simulink model "Glide_slope_model"  (R2020a)
settings: Solver=VariableStepAuto  StartTime=0.0  StopTime=130  RelTol=1e-3
undefined symbols (not defined in the file): med_AA, med_BB, med_CC, med_DD, trim_control_lo
settings Model: Creator=mathi  LastModifiedBy=mathi

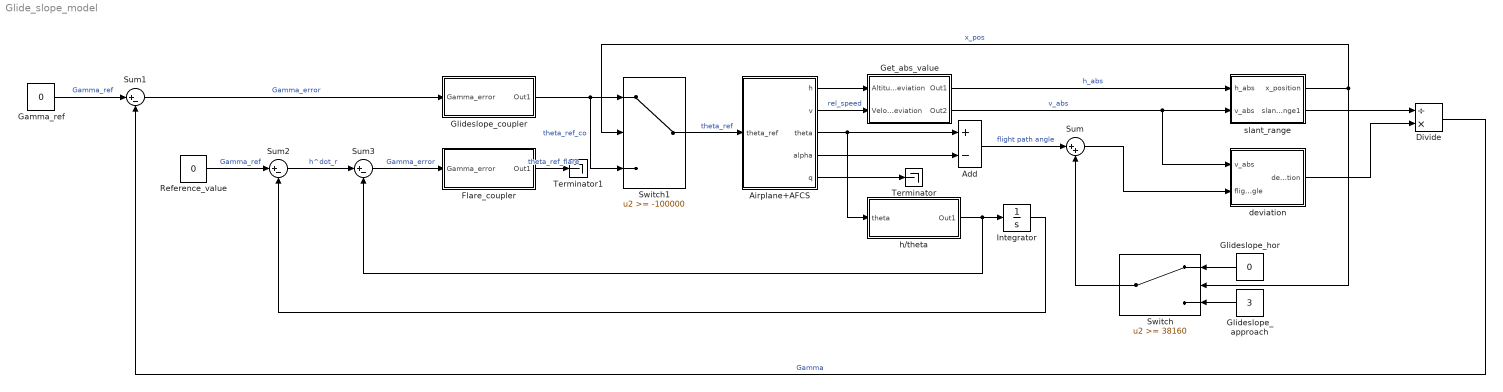
== system Glide_slope_model ==
  Add : Sum  Inputs=+-
  Airplane+AFCS : Subsystem
  Divide : Product  Inputs=/*
  Flare_coupler : Subsystem
  Gamma_ref : Constant  Value=0
  Get_abs_value : Subsystem
  Glideslope_approach : Constant  Value=3
  Glideslope_coupler : Subsystem
  Glideslope_hor : Constant  Value=0
  Integrator : Integrator
  Reference_value : Constant  Value=0
  Sum : Sum  Inputs=|++
  Sum1 : Sum  Inputs=|+-
  Sum2 : Sum  Inputs=|+-
  Sum3 : Sum  Inputs=|+-
  Switch : Switch  Threshold=38160
  Switch1 : Switch  Threshold=-100000
  Terminator : Terminator
  Terminator1 : Terminator
  deviation : Subsystem
  h/theta : Subsystem
  slant_range : Subsystem
  wires:
  Add/1 -> Sum/1  "flight path angle"
  Sum1/1 -> Glideslope_coupler/1(Gamma_error)  "Gamma_error"
  Gamma_ref/1 -> Sum1/1  "Gamma_ref"
  Airplane+AFCS/4(alpha) -> Add/2
  Get_abs_value/2(Out2) -> deviation/1(v_abs), slant_range/2(v_abs)  "v_abs"
  Divide/1 -> Sum1/2  "Gamma"
  Airplane+AFCS/3(theta) -> Add/1, h/theta/1(theta)
  Airplane+AFCS/2(v) -> Get_abs_value/2(Velocity_deviation)  "rel_speed"
  Airplane+AFCS/1(h) -> Get_abs_value/1(Altitude_deviation)
  Airplane+AFCS/5(q) -> Terminator/1
  Get_abs_value/1(Out1) -> slant_range/1(h_abs)  "h_abs"
  Sum/1 -> deviation/2(flight_path_angle)
  deviation/1(deviation) -> Divide/2
  slant_range/2(slant_range1) -> Divide/1
  slant_range/1(x_position) -> Switch1/2, Switch/2  "x_pos"
  Glideslope_approach/1 -> Switch/3
  Glideslope_hor/1 -> Switch/1
  Switch/1 -> Sum/2
  Glideslope_coupler/1(Out1) -> Switch1/3, Switch1/1  "theta_ref_co"
  Switch1/1 -> Airplane+AFCS/1(theta_ref)  "theta_ref"
  Reference_value/1 -> Sum2/1  "Gamma_ref"
  Sum2/1 -> Sum3/1  "h^dot_r"
  Sum3/1 -> Flare_coupler/1(Gamma_error)  "Gamma_error"
  h/theta/1(Out1) -> Sum3/2, Integrator/1
  Integrator/1 -> Sum2/2
  Flare_coupler/1(Out1) -> Terminator1/1  "theta_ref_flare"

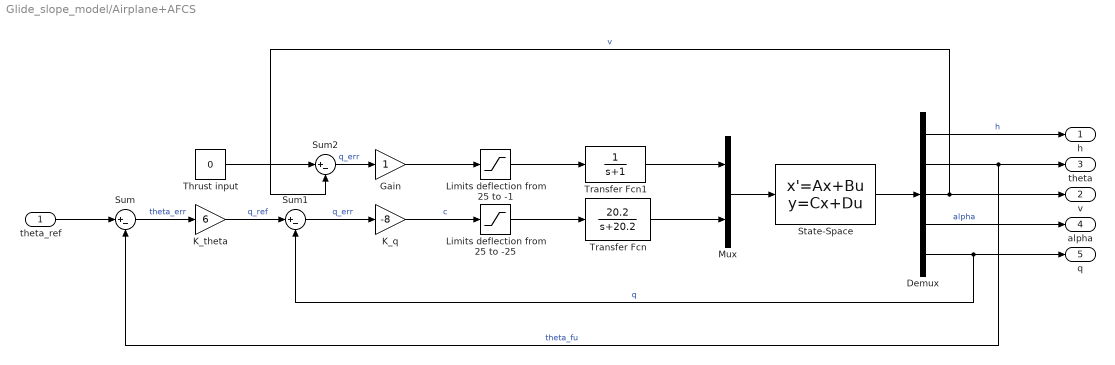
== system Glide_slope_model/Airplane+AFCS ==
  theta_ref : Inport
  Demux : Demux  Outputs=5
  Gain : Gain
  K_q : Gain  Gain=-8
  K_theta : Gain  Gain=6
  Limits deflection from 25 to -1 : Saturate  UpperLimit=25-trim_control_lo(1)  LowerLimit=-25
  Limits deflection from 25 to -25 : Saturate  UpperLimit=25-trim_control_lo(1)  LowerLimit=-25
  Mux : Mux  Inputs=2
  State-Space : StateSpace  A=med_AA  B=med_BB  C=med_CC  D=med_DD  InitialCondition=0
  Sum : Sum  Inputs=|+-
  Sum1 : Sum  Inputs=|+-
  Sum2 : Sum  Inputs=|+-
  Thrust input : Constant  Value=0
  Transfer Fcn : TransferFcn  Numerator=[0 20.2]  Denominator=[1 20.2]
  Transfer Fcn1 : TransferFcn  Denominator=[1 1]
  h : Outport
  v : Outport  Port=2
  theta : Outport  Port=3
  alpha : Outport  Port=4
  q : Outport  Port=5
  wires:
  theta_ref/1 -> Sum/1
  K_theta/1 -> Sum1/1  "q_ref"
  Sum1/1 -> K_q/1  "q_err"
  Mux/1 -> State-Space/1
  Demux/2 -> theta/1, Sum/2  "theta_fu"
  State-Space/1 -> Demux/1
  Demux/5 -> Sum1/2, q/1  "q"
  Demux/4 -> alpha/1  "alpha"
  Demux/3 -> v/1, Sum2/2  "v"
  Demux/1 -> h/1  "h"
  Transfer Fcn/1 -> Mux/2
  K_q/1 -> Limits deflection from 25 to -25/1  "c"
  Limits deflection from 25 to -25/1 -> Transfer Fcn/1
  Sum/1 -> K_theta/1  "theta_err"
  Transfer Fcn1/1 -> Mux/1
  Limits deflection from 25 to -1/1 -> Transfer Fcn1/1
  Gain/1 -> Limits deflection from 25 to -1/1
  Thrust input/1 -> Sum2/1
  Sum2/1 -> Gain/1  "q_err"

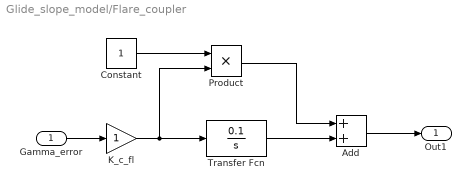
== system Glide_slope_model/Flare_coupler ==
  Gamma_error : Inport
  Add : Sum
  Constant : Constant
  K_c_fl : Gain
  Product : Product
  Transfer Fcn : TransferFcn  Numerator=[0 0.1]  Denominator=[1 0]
  Out1 : Outport
  wires:
  Gamma_error/1 -> K_c_fl/1
  K_c_fl/1 -> Transfer Fcn/1, Product/2
  Constant/1 -> Product/1
  Product/1 -> Add/1
  Add/1 -> Out1/1
  Transfer Fcn/1 -> Add/2

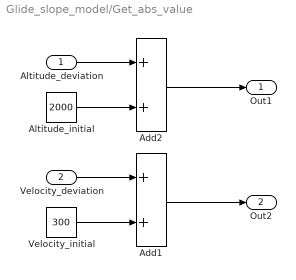
== system Glide_slope_model/Get_abs_value ==
  Altitude_deviation : Inport
  Velocity_deviation : Inport  Port=2
  Add1 : Sum
  Add2 : Sum
  Altitude_initial : Constant  Value=2000
  Velocity_initial : Constant  Value=300
  Out1 : Outport
  Out2 : Outport  Port=2
  wires:
  Velocity_deviation/1 -> Add1/1
  Velocity_initial/1 -> Add1/2
  Add1/1 -> Out2/1
  Altitude_deviation/1 -> Add2/1
  Altitude_initial/1 -> Add2/2
  Add2/1 -> Out1/1

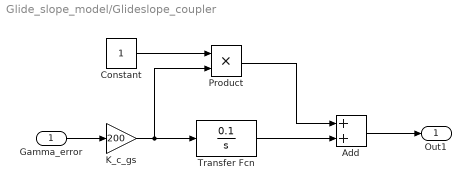
== system Glide_slope_model/Glideslope_coupler ==
  Gamma_error : Inport
  Add : Sum
  Constant : Constant
  K_c_gs : Gain  Gain=200
  Product : Product
  Transfer Fcn : TransferFcn  Numerator=[0 0.1]  Denominator=[1 0]
  Out1 : Outport
  wires:
  Transfer Fcn/1 -> Add/2
  Gamma_error/1 -> K_c_gs/1
  K_c_gs/1 -> Transfer Fcn/1, Product/2
  Constant/1 -> Product/1
  Product/1 -> Add/1
  Add/1 -> Out1/1

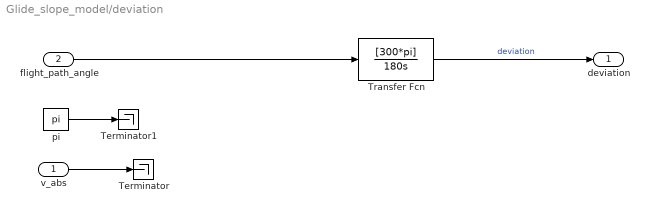
== system Glide_slope_model/deviation ==
  v_abs : Inport
  flight_path_angle : Inport  Port=2
  Terminator : Terminator
  Terminator1 : Terminator
  Transfer Fcn : TransferFcn  Numerator=[300*pi]  Denominator=[180 0]
  pi : Constant  Value=pi
  deviation : Outport
  wires:
  Transfer Fcn/1 -> deviation/1  "deviation"
  flight_path_angle/1 -> Transfer Fcn/1
  v_abs/1 -> Terminator/1
  pi/1 -> Terminator1/1

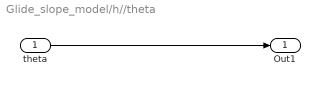
== system Glide_slope_model/h//theta ==
  theta : Inport
  Out1 : Outport
  wires:
  theta/1 -> Out1/1

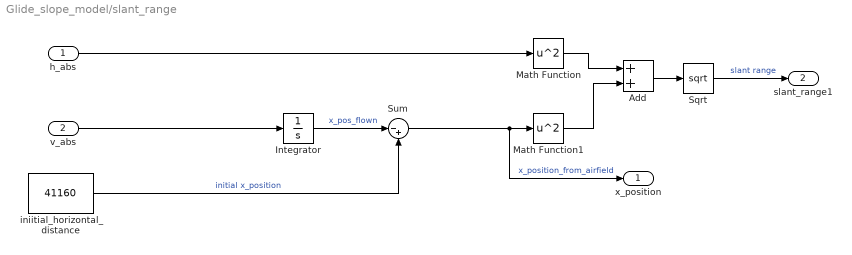
== system Glide_slope_model/slant_range ==
  h_abs : Inport
  v_abs : Inport  Port=2
  Add : Sum
  Integrator : Integrator
  Math Function : Math  Operator=square  SaturateOnIntegerOverflow=on
  Math Function1 : Math  Operator=square  SaturateOnIntegerOverflow=on
  Sqrt : Sqrt  SaturateOnIntegerOverflow=on
  Sum : Sum  Inputs=|-+
  iniitial_horizontal_distance : Constant  Value=41160
  x_position : Outport
  slant_range1 : Outport  Port=2
  wires:
  h_abs/1 -> Math Function/1
  v_abs/1 -> Integrator/1
  iniitial_horizontal_distance/1 -> Sum/2  "initial x_position"
  Integrator/1 -> Sum/1  "x_pos_flown"
  Sum/1 -> x_position/1, Math Function1/1  "x_position_from_airfield"
  Math Function/1 -> Add/1
  Math Function1/1 -> Add/2
  Add/1 -> Sqrt/1
  Sqrt/1 -> slant_range1/1  "slant range"
